simulink model "p3_w3_car_Highway"  (R2023b)
settings: Solver=FixedStepAuto  StartTime=0.0  StopTime=750  FixedStep=0.01  RelTol=1e-3
values from neighbouring files (symbols this model uses):
  HighwayDriveData = [0 ... (first row only)    [initDriveCycle.m]
  HighwayTime = (0:1:765)'    [initDriveCycle.m]
undefined symbols (not defined in the file or in its folder): batData, C0, C1, C2, carData, Iw, M, motorData, mph2mps, r
libraries: slpidlib x1
settings Model: Creator=anshu16  LastModifiedBy=xavie
settings SolverCC: AlgebraicLoopSolver=TrustRegion
settings OptimizationCC: ReuseModelBlockBuffer=off
settings DebuggingCC: UnconnectedInputMsg=warning  UnconnectedOutputMsg=warning  UnconnectedLineMsg=warning
settings ModelReferenceCC: EnableRefExpFcnMdlSchedulingChecks=on
settings SFSimCC: CustomCodeUndefinedFunction=UseInterfaceOnly

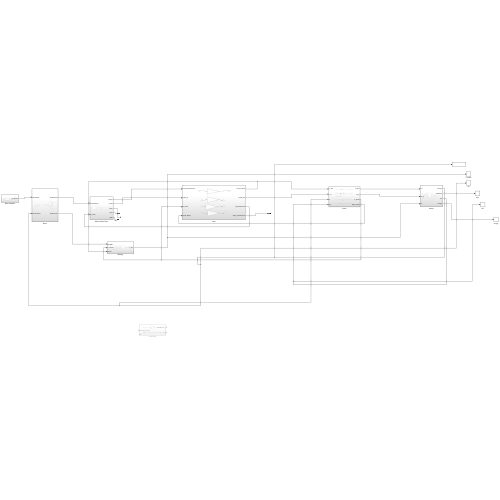
[thumbnail: Simulink's stored preview of the top-level diagram]
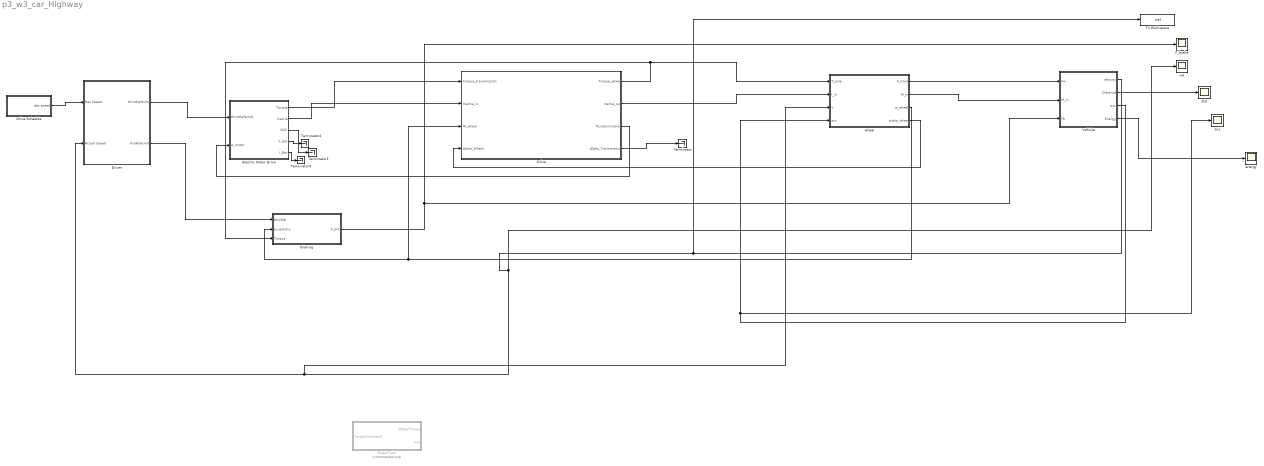
== system p3_w3_car_Highway ==
  " Drive" : Subsystem
  Braking : Subsystem
  Drive Schedule : Subsystem
  "Driver " : Subsystem
  Electric Motor Drive : Subsystem
  F_brake : Scope
  PowerTrain : Subsystem  Commented=on
  Terminator{,1..3} (4 alike) : Terminator
  To Workspace : ToWorkspace  VariableName=vel  SaveFormat=Timeseries  SampleTime=-1
  Vehicle : Subsystem
  acc : Scope
  dist : Scope
  energy : Scope
  vel : Scope
  "wheel " : Subsystem
  wires:
  Drive Schedule/1("des speed ") -> "Driver "/1("Des Speed ")
  "Driver "/2("brake%cmd ") -> Braking/1("BrkCMD ")
  Braking/1("F_brk ") -> F_brake/1, Vehicle/3("Fb ")
  Vehicle/3(acc) -> acc/1, "wheel "/4(acc)
  "wheel "/2(M_in) -> Vehicle/2("M_in ")
  "wheel "/1(F_track) -> Vehicle/1("Fw ")
  Vehicle/2("Distance ") -> dist/1
  Vehicle/1("velocity ") -> vel/1, "wheel "/3(V), "Driver "/2(Actual Speed), To Workspace/1
  "wheel "/4(alpha_wheel) -> " Drive"/4(Alpha_Wheel)
  "wheel "/3(w_wheel) -> Braking/2("w_velocity "), " Drive"/3(W_wheel)
  "Driver "/1(throttle%cmd) -> Electric Motor Drive/1(throttle%cmd)
  Electric Motor Drive/1(Torque) -> " Drive"/1(Torque_transmission)
  Vehicle/4(Energy) -> energy/1
  " Drive"/4(Alpha_Transmission) -> Terminator/1
  " Drive"/1(Torque_wheel) -> Braking/3(Torque), "wheel "/1(T_axle)
  Electric Motor Drive/2(Inertia) -> " Drive"/2(Inertia_in)
  " Drive"/2(Inertia_out) -> "wheel "/2(I_in)
  " Drive"/3(W_transmission) -> Electric Motor Drive/2(w_motor)
  Electric Motor Drive/3(SOC) -> Terminator1/1
  Electric Motor Drive/4(V_bat) -> Terminator2/1
  Electric Motor Drive/5(I_Bat) -> Terminator3/1

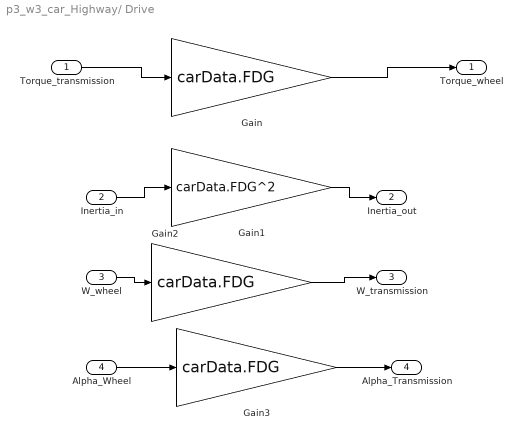
== system p3_w3_car_Highway/ Drive ==
  Torque_transmission : Inport
  Inertia_in : Inport  Port=2
  W_wheel : Inport  Port=3
  Alpha_Wheel : Inport  Port=4
  Gain : Gain  Gain=carData.FDG
  Gain1 : Gain  Gain=carData.FDG^2
  Gain2 : Gain  Gain=carData.FDG
  Gain3 : Gain  Gain=carData.FDG
  Torque_wheel : Outport
  Inertia_out : Outport  Port=2
  W_transmission : Outport  Port=3
  Alpha_Transmission : Outport  Port=4
  wires:
  Torque_transmission/1 -> Gain/1
  Inertia_in/1 -> Gain1/1
  W_wheel/1 -> Gain2/1
  Alpha_Wheel/1 -> Gain3/1
  Gain/1 -> Torque_wheel/1
  Gain1/1 -> Inertia_out/1
  Gain2/1 -> W_transmission/1
  Gain3/1 -> Alpha_Transmission/1

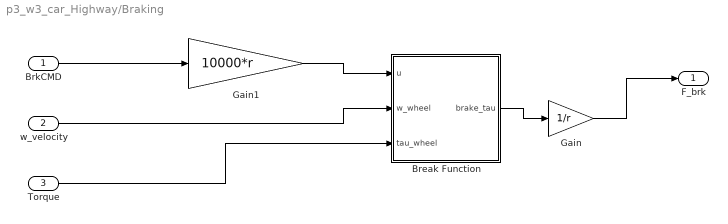
== system p3_w3_car_Highway/Braking ==
  "BrkCMD " : Inport
  "w_velocity " : Inport  Port=2
  Torque : Inport  Port=3
  Break Function : MATLAB Function  TreatAsAtomicUnit=on
  Gain : Gain  Gain=1/r
  Gain1 : Gain  Gain=10000*r
  "F_brk " : Outport  VectorParamsAs1DForOutWhenUnconnected=off
  wires:
  "BrkCMD "/1 -> Gain1/1
  Gain1/1 -> Break Function/1(u)
  "w_velocity "/1 -> Break Function/2(w_wheel)
  Break Function/1(brake_tau) -> Gain/1
  Torque/1 -> Break Function/3(tau_wheel)
  Gain/1 -> "F_brk "/1

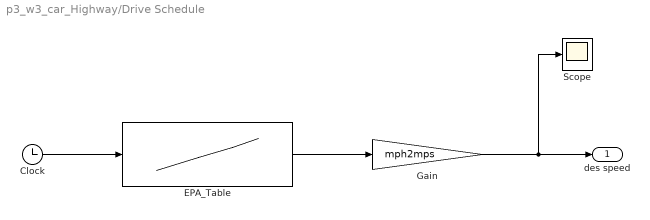
== system p3_w3_car_Highway/Drive Schedule ==
  Clock : Clock
  EPA_Table : Lookup_n-D  NumberOfTableDimensions=1  BreakpointsForDimension1=HighwayTime  Table=HighwayDriveData  InternalRulePriority=Speed  RndMeth=Simplest
  Gain : Gain  Gain=mph2mps
  Scope : Scope
  "des speed " : Outport  VectorParamsAs1DForOutWhenUnconnected=off
  wires:
  Clock/1 -> EPA_Table/1
  EPA_Table/1 -> Gain/1
  Gain/1 -> "des speed "/1, Scope/1

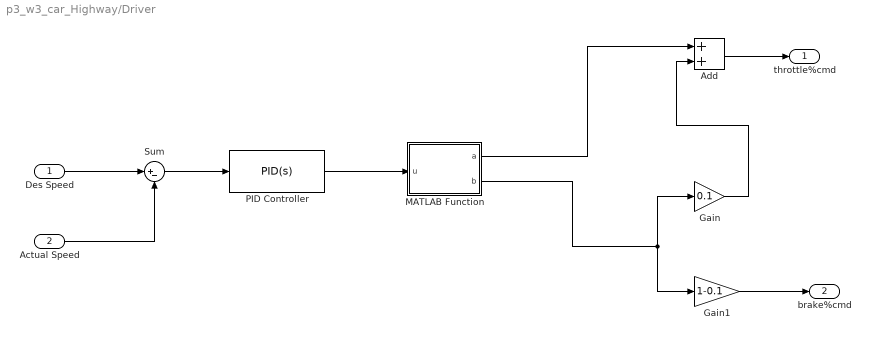
== system p3_w3_car_Highway/Driver  ==
  "Des Speed " : Inport
  Actual Speed : Inport  Port=2
  Add : Sum
  Gain : Gain  Gain=0.1
  Gain1 : Gain  Gain=1-0.1
  MATLAB Function : MATLAB Function  TreatAsAtomicUnit=on
  PID Controller : slpidlib/PID Controller  Controller=PID  Form=Parallel  TimeDomain=Continuous-time  UseExternalTs=off  SampleTime=-1  IntegratorMethod=Forward Euler  FilterMethod=Forward Euler  ControllerParametersSource=internal  P=0.1  I=0  UseKiTs=off  D=0  N=100  UseFilter=on  TunerSelectOption=Transfer Function Based (PID Tuner App)  InitialConditionSource=internal  InitialConditionForIntegrator=0  InitialConditionForFilter=0  DifferentiatorICPrevScaledInput=0  ExternalReset=none  TrackingMode=off  Kt=1  LimitOutput=on  SatLimitsSource=internal  UpperSaturationLimit=1  LowerSaturationLimit=-1  LinearizeAsGain=off  AntiWindupMode=none  Kb=1  LimitIntegrator=off  UpperIntegratorSaturationLimit=inf  LowerIntegratorSaturationLimit=-inf  POutMin=[]  POutMax=[]  IOutMin=[]  IOutMax=[]  DOutMin=[]  DOutMax=[]  NOutMin=[]  NOutMax=[]  SumOutMin=[]  SumOutMax=[]  SaturationOutMin=[]  SaturationOutMax=[]  PParamMin=[]  PParamMax=[]  IParamMin=[]  IParamMax=[]  DParamMin=[]  DParamMax=[]  NParamMin=[]  NParamMax=[]  KbParamMin=[]  KbParamMax=[]  KtParamMin=[]  KtParamMax=[]  KbOutMin=[]  KbOutMax=[]  KtOutMin=[]  KtOutMax=[]  IntegratorOutMin=[]  IntegratorOutMax=[]  FilterOutMin=[]  FilterOutMax=[]  SumI1OutMin=[]  SumI1OutMax=[]  SumI2OutMin=[]  SumI2OutMax=[]  SumI3OutMin=[]  SumI3OutMax=[]  SumI4OutMin=[]  SumI4OutMax=[]  SumDOutMin=[]  SumDOutMax=[]  DifferentiatorOutMin=[]  DifferentiatorOutMax=[]  FilterDiffOutCoefMin=[]  FilterDiffOutCoefMax=[]  ReciprocalOutMin=[]  ReciprocalOutMax=[]  SumDenOutMin=[]  SumDenOutMax=[]  SumNumOutMin=[]  SumNumOutMax=[]  DivideOutMin=[]  DivideOutMax=[]  UdiffTsProdOutMin=[]  UdiffTsProdOutMax=[]  NTsProdOutMin=[]  NTsProdOutMax=[]  UintegralTsProdOutMin=[]  UintegralTsProdOutMax=[]  UngainTsProdOutMin=[]  UngainTsProdOutMax=[]  ClampingZeroOutDataTypeStr=Inherit: Inherit via back propagation  ClampingZeroOutMin=[]  ClampingZeroOutMax=[]  FilterDenConstantOutDataTypeStr=Inherit: Inherit via back propagation  FilterDenConstantOutMin=[]  FilterDenConstantOutMax=[]  PCopyOutDataTypeStr=Inherit: Inherit via back propagation  PCopyOutMin=[]  PCopyOutMax=[]  NCopyOutDataTypeStr=Inherit: Inherit via back propagation  NCopyOutMin=[]  NCopyOutMax=[]  IntegratorContinuousStateAttributes=''  IntegratorStateMustResolveToSignalObject=off  IntegratorRTWStateStorageClass=Auto  FilterContinuousStateAttributes=''  FilterStateMustResolveToSignalObject=off  FilterRTWStateStorageClass=Auto  ParallelPVariant=InternalParameters  IdealPVariant=Disabled  IVariant=InternalParameters  DVariant=InternalParameters  IntegratorVariant=Continuous  SatVariant=Enabled  AWVariant=Passthrough  PCopyVariant=Disabled  TRVariant=Disabled  FdbkBlocksVariant=Forward  IdealPFdbkVariant=Disabled  SatFdbkVariant=Disabled  DerivativeFilterVariant=ContFilter  NVariant=InternalParameters  NCopyVariant=Disabled  FilterICVariant=InternalICsFilter  IntegratorICVariant=InternalICs  ExternalResetVariant=Disabled  TRSumVariant=Passthrough  SumFdbkVariant=Disabled  SumVariant=Sum_PID  TsampFilterVariant=InternalTs  TsampNgainVariant=Passthrough  TsampIntegralVariant=Disabled_SignalSpec  ExternalSaturationOutDataTypeStr=Inherit: Same as second input
  Sum : Sum  Inputs=|+-
  throttle%cmd : Outport
  "brake%cmd " : Outport  Port=2
  wires:
  "Des Speed "/1 -> Sum/1
  Actual Speed/1 -> Sum/2
  MATLAB Function/2(b) -> Gain/1, Gain1/1
  Sum/1 -> PID Controller/1
  PID Controller/1 -> MATLAB Function/1(u)
  Gain/1 -> Add/2
  MATLAB Function/1(a) -> Add/1
  Add/1 -> throttle%cmd/1
  Gain1/1 -> "brake%cmd "/1

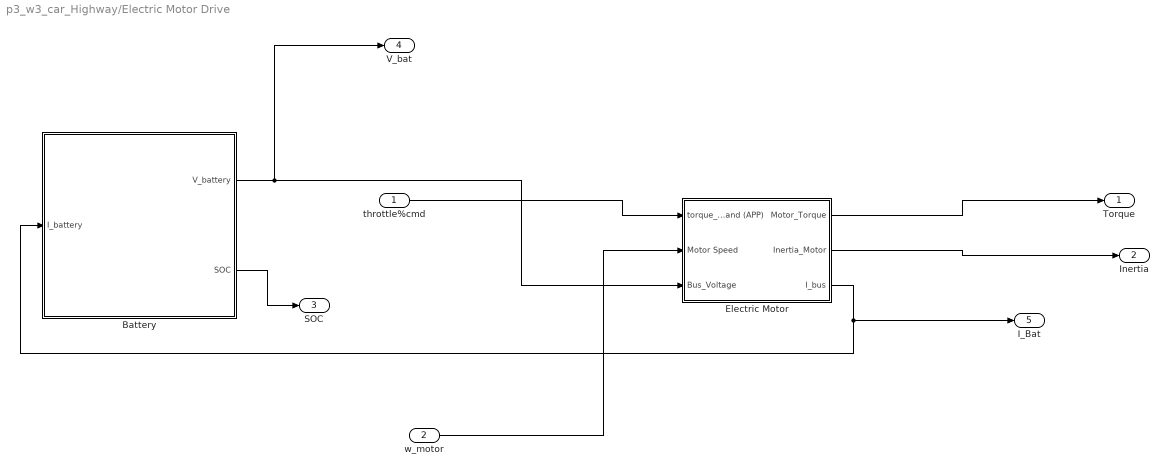
== system p3_w3_car_Highway/Electric Motor Drive ==
  throttle%cmd : Inport
  w_motor : Inport  Port=2
  Battery : Subsystem
  Electric Motor : Subsystem
  Torque : Outport
  Inertia : Outport  Port=2
  SOC : Outport  Port=3
  V_bat : Outport  Port=4
  I_Bat : Outport  Port=5
  wires:
  throttle%cmd/1 -> Electric Motor/1(torque_command (APP))
  Electric Motor/1(Motor_Torque) -> Torque/1
  Electric Motor/2(Inertia_Motor) -> Inertia/1
  w_motor/1 -> Electric Motor/2(Motor Speed)
  Battery/1(V_battery) -> V_bat/1, Electric Motor/3(Bus_Voltage)
  Battery/2(SOC) -> SOC/1
  Electric Motor/3(I_bus) -> I_Bat/1, Battery/1(I_battery)

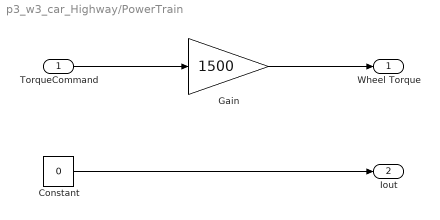
== system p3_w3_car_Highway/PowerTrain ==
  TorqueCommand : Inport
  Constant : Constant  Value=0
  Gain : Gain  Gain=1500
  Wheel Torque : Outport
  Iout : Outport  Port=2
  wires:
  TorqueCommand/1 -> Gain/1
  Gain/1 -> Wheel Torque/1
  Constant/1 -> Iout/1

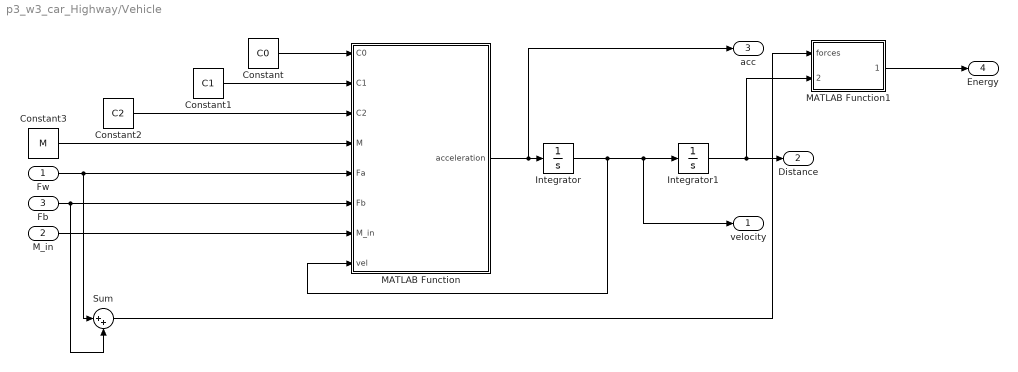
== system p3_w3_car_Highway/Vehicle ==
  "Fw " : Inport
  "M_in " : Inport  Port=2
  "Fb " : Inport  Port=3
  Constant : Constant  Value=C0
  Constant1 : Constant  Value=C1
  Constant2 : Constant  Value=C2
  Constant3 : Constant  Value=M
  Integrator : Integrator  LimitOutput=on  LowerSaturationLimit=0
  Integrator1 : Integrator
  MATLAB Function : MATLAB Function  TreatAsAtomicUnit=on
  MATLAB Function1 : MATLAB Function  TreatAsAtomicUnit=on
  Sum : Sum  Inputs=|++
  "velocity " : Outport  VectorParamsAs1DForOutWhenUnconnected=off
  "Distance " : Outport  Port=2  VectorParamsAs1DForOutWhenUnconnected=off
  acc : Outport  Port=3
  Energy : Outport  Port=4  VectorParamsAs1DForOutWhenUnconnected=off
  wires:
  Constant1/1 -> MATLAB Function/2(C1)
  Constant/1 -> MATLAB Function/1(C0)
  MATLAB Function/1(acceleration) -> acc/1, Integrator/1
  Constant2/1 -> MATLAB Function/3(C2)
  Constant3/1 -> MATLAB Function/4(M)
  "Fw "/1 -> Sum/1, MATLAB Function/5(Fa)
  "Fb "/1 -> MATLAB Function/6(Fb), Sum/2
  Integrator/1 -> MATLAB Function/8(vel), "velocity "/1, Integrator1/1
  Integrator1/1 -> MATLAB Function1/2(distance), "Distance "/1
  "M_in "/1 -> MATLAB Function/7(M_in)
  Sum/1 -> MATLAB Function1/1(forces)
  MATLAB Function1/1(energy) -> Energy/1

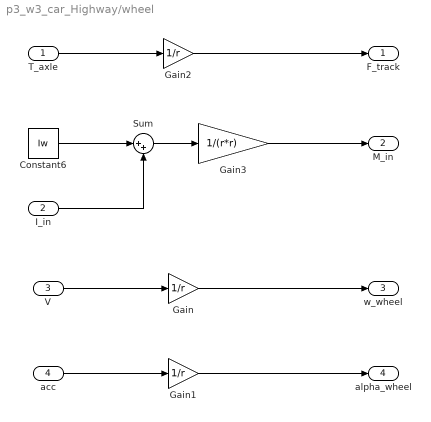
== system p3_w3_car_Highway/wheel  ==
  T_axle : Inport
  I_in : Inport  Port=2
  V : Inport  Port=3
  acc : Inport  Port=4
  Constant6 : Constant  Value=Iw
  Gain : Gain  Gain=1/r
  Gain1 : Gain  Gain=1/r
  Gain2 : Gain  Gain=1/r
  Gain3 : Gain  Gain=1/(r*r)
  Sum : Sum  Inputs=|++
  F_track : Outport
  M_in : Outport  Port=2
  w_wheel : Outport  Port=3
  alpha_wheel : Outport  Port=4
  wires:
  Gain/1 -> w_wheel/1
  V/1 -> Gain/1
  acc/1 -> Gain1/1
  Gain1/1 -> alpha_wheel/1
  T_axle/1 -> Gain2/1
  Gain2/1 -> F_track/1
  Gain3/1 -> M_in/1
  Constant6/1 -> Sum/1
  I_in/1 -> Sum/2
  Sum/1 -> Gain3/1

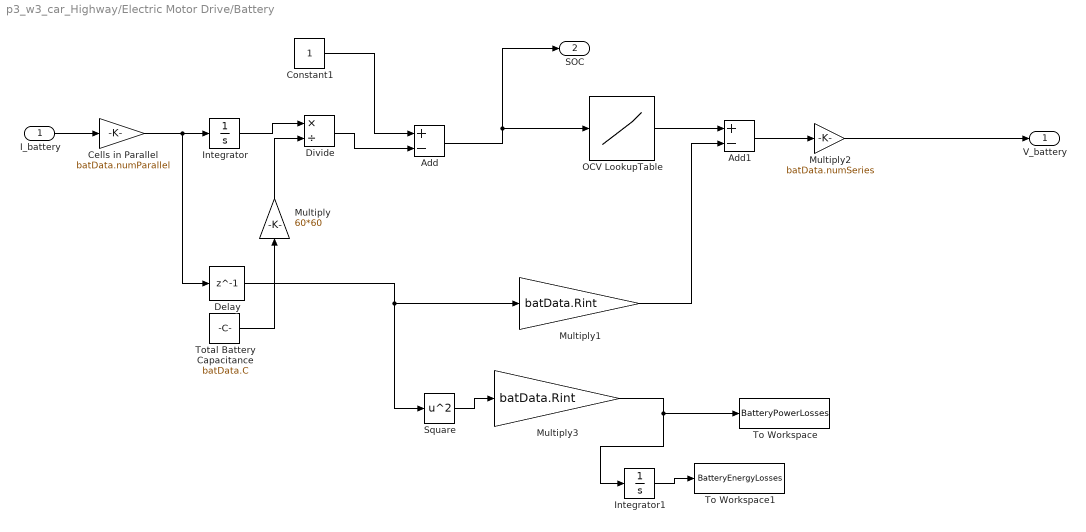
== system p3_w3_car_Highway/Electric Motor Drive/Battery ==
  I_battery : Inport
  Add : Sum  Inputs=+-
  Add1 : Sum  Inputs=+-
  Cells in Parallel : Gain  Gain=batData.numParallel
  Constant1 : Constant
  Delay : Delay  DelayLength=1
  Divide : Product  Inputs=*/
  Integrator : Integrator
  Integrator1 : Integrator
  Multiply : Gain  Gain=60*60
  Multiply1 : Gain  Gain=batData.Rint
  Multiply2 : Gain  Gain=batData.numSeries
  Multiply3 : Gain  Gain=batData.Rint
  OCV LookupTable : Lookup_n-D  NumberOfTableDimensions=1  BreakpointsForDimension1=batData.SOC  Table=batData.OCV  InternalRulePriority=Speed  RndMeth=Simplest
  Square : Math  Operator=square
  To Workspace : ToWorkspace  VariableName=BatteryPowerLosses  SaveFormat=Timeseries  SampleTime=-1
  To Workspace1 : ToWorkspace  VariableName=BatteryEnergyLosses  SaveFormat=Timeseries  SampleTime=-1
  Total Battery Capacitance : Constant  Value=batData.C
  V_battery : Outport
  SOC : Outport  Port=2
  wires:
  I_battery/1 -> Cells in Parallel/1
  Multiply2/1 -> V_battery/1
  Cells in Parallel/1 -> Delay/1, Integrator/1
  Integrator/1 -> Divide/1
  Constant1/1 -> Add/1
  Divide/1 -> Add/2
  Add/1 -> OCV LookupTable/1, SOC/1
  OCV LookupTable/1 -> Add1/1
  Delay/1 -> Square/1, Multiply1/1
  Multiply1/1 -> Add1/2
  Add1/1 -> Multiply2/1
  Multiply3/1 -> To Workspace/1, Integrator1/1
  Square/1 -> Multiply3/1
  Total Battery Capacitance/1 -> Multiply/1
  Integrator1/1 -> To Workspace1/1
  Multiply/1 -> Divide/2

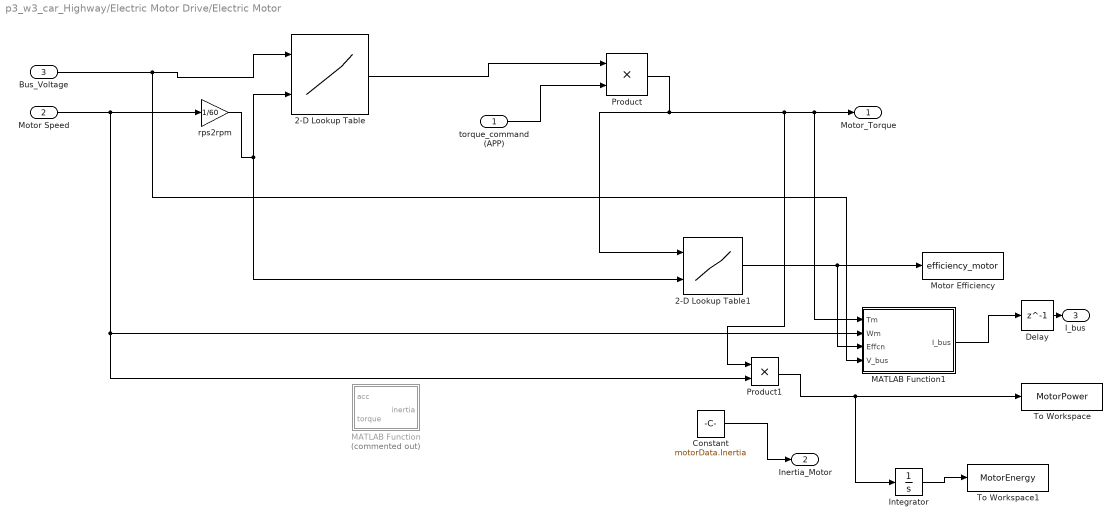
== system p3_w3_car_Highway/Electric Motor Drive/Electric Motor ==
  torque_command (APP) : Inport
  Motor Speed : Inport  Port=2
  Bus_Voltage : Inport  Port=3
  2-D Lookup Table : Lookup_n-D  BreakpointsForDimension1=motorData.vbus  BreakpointsForDimension2=motorData.rpm  Table=motorData.maxtorque  InternalRulePriority=Speed  RndMeth=Simplest
      settings: InputPortMap=u0,u1
  2-D Lookup Table1 : Lookup_n-D  BreakpointsForDimension1=motorData.eta_torque  BreakpointsForDimension2=motorData.eta_speed  Table=motorData.eta_val  InternalRulePriority=Speed  RndMeth=Simplest
      settings: InputPortMap=u0,u1
  Constant : Constant  Value=motorData.Inertia
  Delay : Delay  DelayLength=1
  Integrator : Integrator
  MATLAB Function : MATLAB Function  Commented=on  TreatAsAtomicUnit=on
  MATLAB Function1 : MATLAB Function  TreatAsAtomicUnit=on
  Motor Efficiency : ToWorkspace  VariableName=efficiency_motor  SaveFormat=Timeseries  SampleTime=-1
  Product : Product
  Product1 : Product
  To Workspace : ToWorkspace  VariableName=MotorPower  SaveFormat=Timeseries  SampleTime=-1
  To Workspace1 : ToWorkspace  VariableName=MotorEnergy  SaveFormat=Timeseries  SampleTime=-1
  rps2rpm : Gain  Gain=1/60
  Motor_Torque : Outport
  Inertia_Motor : Outport  Port=2
  I_bus : Outport  Port=3
  wires:
  Motor Speed/1 -> MATLAB Function1/2(Wm), Product1/2, rps2rpm/1
  rps2rpm/1 -> 2-D Lookup Table1/2, 2-D Lookup Table/2
  2-D Lookup Table/1 -> Product/1
  torque_command (APP)/1 -> Product/2
  Product/1 -> 2-D Lookup Table1/1, Product1/1, MATLAB Function1/1(Tm), Motor_Torque/1
  Bus_Voltage/1 -> MATLAB Function1/4(V_bus), 2-D Lookup Table/1
  2-D Lookup Table1/1 -> MATLAB Function1/3(Effcn), Motor Efficiency/1
  Constant/1 -> Inertia_Motor/1
  Product1/1 -> Integrator/1, To Workspace/1
  Integrator/1 -> To Workspace1/1
  Delay/1 -> I_bus/1
  MATLAB Function1/1(I_bus) -> Delay/1

== matlab function p3_w3_car_Highway/Driver /MATLAB Function ==
  data: u input; a output; b output
% Checks if there is a difference between actual speed and desired speed

% u is calculated using the sum function in the simulink model

function [a,b] = fcn(u)

if u>0 % If the difference is greater than zero, then we need to speed up since actual speed is less than desired speed
    acc=u; % We send how much we need to speed up to the throttle command
    brk=0; % Do nothing for the break command
elseif u<0 % If the difference is less than zero, then we need to slow down since the actual speed is less than the desired speed
    acc=0; % Do nothing for throttle command
    brk=-u; % We send how much we need to break to the break command
else % If the desired and actual speed is the same
    acc=0; % Do nothing for throttle command
    brk=0; % Do nothing for the break command
end
a= acc; % storing how much acceleration required to a
b= brk; % storing how much break acceleration required to b

== matlab function p3_w3_car_Highway/Vehicle/MATLAB Function ==
  data: C0 input; acceleration output; C1 input; C2 input; M input; Fa input; Fb input; M_in input; vel input
function acceleration   = vehicle(C0,C1,C2,M,Fa,Fb,M_in, vel)

acceleration = (((Fa-Fb))-(C0+ C1*vel + C2*(vel)^2))/(M+M_in);

== matlab function p3_w3_car_Highway/Vehicle/MATLAB Function1 ==
  data: forces input; energy output; distance input
function energy = fcn(forces, distance)

energy = dot(forces, distance);

== matlab function p3_w3_car_Highway/Electric Motor Drive/Electric Motor/MATLAB Function ==
  data: acc input; inertia output; torque input
function inertia= fcn(acc, torque)

inertia = torque/acc;

== matlab function p3_w3_car_Highway/Electric Motor Drive/Electric Motor/MATLAB Function1 ==
  data: Tm input; I_bus output; Wm input; Effcn input; V_bus input
function I_bus = fcn(Tm, Wm, Effcn, V_bus)

Pm = Tm * Wm;
sgn_Pm = Pm/(abs(Pm)+0.001);
Pe = Pm * Effcn^(sgn_Pm); 
I_bus = Pe/V_bus; % Calculating I_bus

== matlab function p3_w3_car_Highway/Braking/Break Function ==
  data: u input; brake_tau output; w_wheel input; tau_wheel input
% Gets the value for the break required as u
% w_wheel is the angular velocity of the wheel
% tau_wheel is the torque of the wheel
% Need to determine whether we use the angular velocity or the actual
% velocity/torque

function brake_tau = fcn(u,w_wheel, tau_wheel)

%y =u*sign(v)

if w_wheel == 0
    brake_tau = -min(abs(tau_wheel), u) * (tau_wheel/(abs(tau_wheel) + 0.001)); % Using sgn approximation if the wheel is not moving
else
    brake_tau = u * (w_wheel/(abs(w_wheel) + 0.001)); % using sgn approximation brake torque if it is moving or reversing (+ve or -ve)
end

% y = u * v/(abs(v)+0.001);
% y = u;
